simulink model "twilio_task"  (Simulink 3.00)
undefined symbols (not defined in the file): application, form, json, Messages, urlencoded, www, x
libraries: stringlib x7, speclib x1, genlib x1

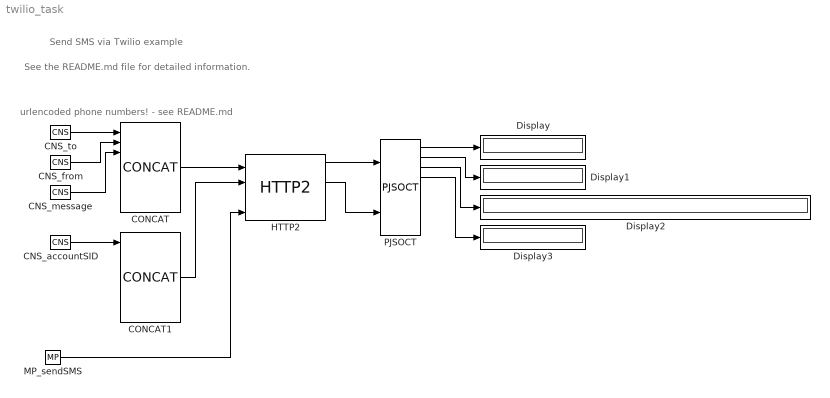
== system twilio_task ==
  note: See the README.md file for detailed information.
  note: urlencoded phone numbers! - see README.md
  note: Send SMS via Twilio example
  CNS_accountSID : stringlib/CNS  scv=YourTwilioAccountSID  nmax=0
  CNS_from : stringlib/CNS  scv=%2B15005550006  nmax=0
  CNS_message : stringlib/CNS  scv=Hello from REXYGEN!  nmax=0
  CNS_to : stringlib/CNS  scv=%2B15005550006  nmax=0
  CONCAT : stringlib/CONCAT  ptrn=To=%1&From=%2&Body=%3  nmax=0
  CONCAT1 : stringlib/CONCAT  ptrn=%1/Messages.json  nmax=0
  Display{,1..3} (4 alike) : Display
      settings: Format=Best fit
  HTTP2 : speclib/HTTP2  url=https://api.twilio.com/2010-04-01/Accounts/  method=2: POST  user=YourTwilioAccountSID  password=YourTwilioAuthToken  VERIFY=off  postmime=application/x-www-form-urlencoded  acceptmime=application/json  timeout=5  BLOCKING=off  nmax=0  postmax=2560  datamax=10240
  MP_sendSMS : genlib/MP  BSTATE=off  pwidth=1  RPTF=off
  PJSOCT : stringlib/PJSOCT  name1=to  name2=from  name3=body  name4=status  nmax=0
  wires:
  CNS_accountSID/1 -> CONCAT1/1
  CNS_from/1 -> CONCAT/2
  CNS_message/1 -> CONCAT/3
  CNS_to/1 -> CONCAT/1
  CONCAT/1 -> HTTP2/1
  CONCAT1/1 -> HTTP2/2
  HTTP2/1 -> PJSOCT/1
  HTTP2/3 -> PJSOCT/2
  MP_sendSMS/1 -> HTTP2/4
  PJSOCT/1 -> Display/1
  PJSOCT/2 -> Display1/1
  PJSOCT/3 -> Display2/1
  PJSOCT/4 -> Display3/1
